simulink model "es2"  (R2020b)
settings: Solver=VariableStepAuto  StartTime=0.0  StopTime=20  MaxStep=0.001  RelTol=1e-3
values from neighbouring files (symbols this model uses):
  c = 0    [ex 5 residual solution.m]
  k = 100    [ex 5 residual solution.m]
  m = 2    [ex 5 residual solution.m]
settings Model: Creator=EREN  LastModifiedBy=drart

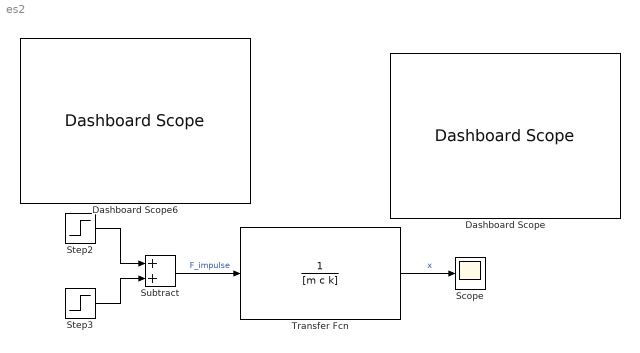
== system es2 ==
  Dashboard Scope : DashboardScope
  Dashboard Scope6 : DashboardScope
  Scope : Scope
  Step2 : Step  Time=0  SampleTime=0
  Step3 : Step  Time=0.01  After=-1  SampleTime=0
  Subtract : Sum
  Transfer Fcn : TransferFcn  Denominator=[m c k]
  wires:
  Transfer Fcn/1 -> Scope/1  "x"
  Subtract/1 -> Transfer Fcn/1  "F_impulse"
  Step2/1 -> Subtract/1
  Step3/1 -> Subtract/2
